simulink model "exercise4_SIM"  (R2025b)
settings: Solver=ode23s  StartTime=0.0  StopTime=p.tend  RelTol=1e-3
values from neighbouring files (symbols this model uses):
  p =     [LoopController.mat]
libraries: cstblocks x1
settings Model: Creator=aless  LastModifiedBy=aless

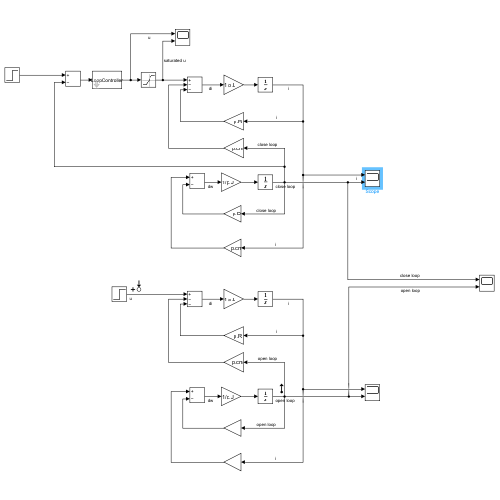
[thumbnail: Simulink's stored preview of the top-level diagram]
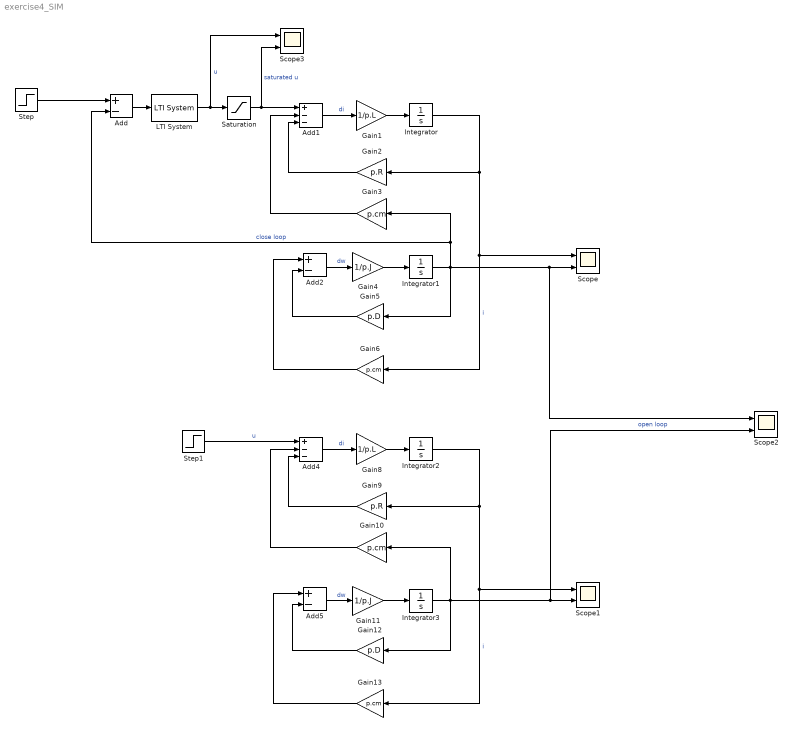
== system exercise4_SIM ==
  Add : Sum  Inputs=+-
  Add1 : Sum  Inputs=+--
  Add2 : Sum  Inputs=+-
  Add4 : Sum  Inputs=+--
  Add5 : Sum  Inputs=+-
  Gain1 : Gain  Gain=1/p.L
  Gain{3,6,10,13} (4 alike) : Gain  Gain=p.cm
  Gain11 : Gain  Gain=1/p.J
  Gain12 : Gain  Gain=p.D
  Gain2 : Gain  Gain=p.R
  Gain4 : Gain  Gain=1/p.J
  Gain5 : Gain  Gain=p.D
  Gain8 : Gain  Gain=1/p.L
  Gain9 : Gain  Gain=p.R
  Integrator{,1..3} (4 alike) : Integrator
  LTI System : cstblocks/LTI System  sys=LoopController  IC=[]  PadeOrder=0
  Saturation : Saturate  UpperLimit=12  LowerLimit=-12
  Scope{,1..3} (4 alike) : Scope  NumInputPorts=2
      Scope settings: ActiveDisplayYMinimum=-0.12942705193551488  ActiveDisplayYMaximum=1.1575895944478998  DataLoggingVariableName=closeLoop
      Scope1 settings: ActiveDisplayYMinimum=-5.2454509775140625  ActiveDisplayYMaximum=47.209058797626568  DataLoggingVariableName=openLoop
      Scope2 settings: ActiveDisplayYMinimum=-1  ActiveDisplayYMaximum=1
      Scope3 settings: ActiveDisplayYMinimum=-1  ActiveDisplayYMaximum=1
  Step : Step  Time=p.t0  After=p.u  SampleTime=0
  Step1 : Step  Time=p.t0  After=p.u  SampleTime=0
  wires:
  Add1/1 -> Gain1/1  "di"
  Gain1/1 -> Integrator/1
  Integrator/1 -> Gain2/1, Gain6/1, Scope/1  "i"
  Gain2/1 -> Add1/3
  Gain3/1 -> Add1/2
  Gain4/1 -> Integrator1/1
  Add2/1 -> Gain4/1  "dw"
  Integrator1/1 -> Gain5/1, Scope2/1, Scope/2, Add/2, Gain3/1  "close loop"
  Gain5/1 -> Add2/2
  Gain6/1 -> Add2/1
  Gain11/1 -> Integrator3/1
  Add5/1 -> Gain11/1  "dw"
  Gain9/1 -> Add4/3
  Gain10/1 -> Add4/2
  Integrator2/1 -> Gain9/1, Gain13/1, Scope1/1  "i"
  Gain13/1 -> Add5/1
  Gain8/1 -> Integrator2/1
  Add4/1 -> Gain8/1  "di"
  Gain12/1 -> Add5/2
  Step1/1 -> Add4/1  "u"
  Integrator3/1 -> Gain12/1, Scope2/2, Scope1/2, Gain10/1  "open loop"
  Step/1 -> Add/1
  Add/1 -> LTI System/1
  LTI System/1 -> Scope3/1, Saturation/1  "u"
  Saturation/1 -> Scope3/2, Add1/1  "saturated u"
